simulink model "BLAC0_ControlloVelocitaNonCompensato"  (R2018b)
settings: Solver=ode1  StartTime=0.0  StopTime=0.1  FixedStep=1e-4  RelTol=1e-3
values from neighbouring files (symbols this model uses):
  B = 3.8e-005    (= 3.8e-05)    [BLAC0_v1.m]    (also in BLAC1_v1.m = 0; BLAC1_v2.m = 0; CAE_11_v_1.m = 0; CAE_14_v1.M = 0)
  J = 0.0000251    (= 2.51e-05)    [BLAC0_v1.m]    (also in BLAC1_v1.m = 0.001; BLAC1_v2.m = 0.001; CAE_11_v_1.m = 0.001; CAE_14_v1.M = 0.001)
  Kc = ms*np*lambdaf/2    (= 0.27)    [BLAC0_v1.m]    (also in BLAC1_v1.m = 0.6; BLAC1_v2.m = 0.6; CAE_11_v_1.m = 0.6; CAE_14_v1.M = 0.6)
  Lsd = 0.005/2    (= 0.0025)    [BLAC0_v1.m]    (also in BLAC1_v1.m = 0.005; BLAC1_v2.m = 0.005; CAE_11_v_1.m = 0.005; CAE_14_v1.M = 0.005)
  Lsq = Lsd    (= 0.0025)    [BLAC0_v1.m]    (also in BLAC1_v1.m = 0.005; BLAC1_v2.m = 0.005; CAE_11_v_1.m = 0.005; CAE_14_v1.M = 0.005)
  np = 2    [BLAC0_v1.m]    (also in BLAC1_v1.m = 4; BLAC1_v2.m = 4; CAE_11_v_1.m = 4; CAE_14_v1.M = 4)
  PSIPM = lambdaf    (= 0.09)    [BLAC0_v1.m]
  Rs = 3.1/2    (= 1.55)    [BLAC0_v1.m]    (also in BLAC1_v1.m = 1; BLAC1_v2.m = 1; CAE_11_v_1.m = 1; CAE_14_v1.M = 1)
  wrr = 1256.6    [BLAC0_v1.m]    (also in BLAC1_v1.m = 300; BLAC1_v2.m = 300)
settings Model: Creator=franc  LastModifiedBy=anton

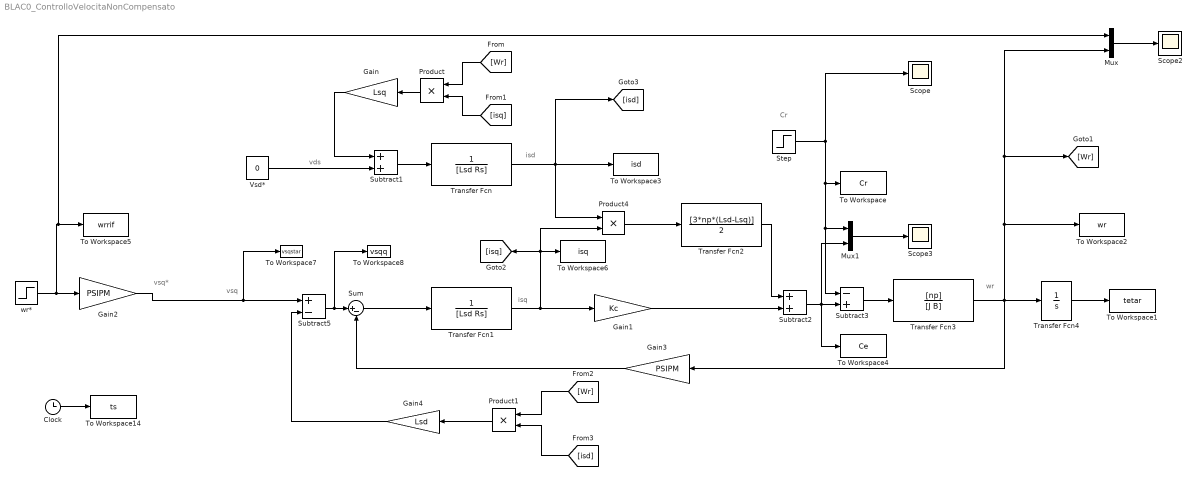
== system BLAC0_ControlloVelocitaNonCompensato ==
  note: isd
  note: isq
  note: wr
  note: vsq
  note: vsq*
  note: Cr
  note: vds
  Clock : Clock
  Gain : Gain  Gain=Lsq
  Gain1 : Gain  Gain=Kc
  Gain2 : Gain  Gain=PSIPM
  Gain3 : Gain  Gain=PSIPM
  Gain4 : Gain  Gain=Lsd
  Mux : Mux  Inputs=2
  Mux1 : Mux  Inputs=2
  Product : Product
  Product1 : Product
  Product4 : Product
  Scope : Scope
  Scope2 : Scope
  Scope3 : Scope
  Step : Step  Time=0.05  After=0.6  SampleTime=0
  Subtract1 : Sum
  Subtract2 : Sum
  Subtract3 : Sum  Inputs=-+
  Subtract5 : Sum  Inputs=+-
  Sum : Sum  Inputs=|+-
  To Workspace : ToWorkspace  VariableName=Cr  SampleTime=-1
  To Workspace1 : ToWorkspace  VariableName=tetar  SaveFormat=Timeseries  SampleTime=-1
  To Workspace14 : ToWorkspace  VariableName=ts  SampleTime=-1
  To Workspace2 : ToWorkspace  VariableName=wr  SampleTime=-1
  To Workspace3 : ToWorkspace  VariableName=isd  SaveFormat=Timeseries  SampleTime=-1
  To Workspace4 : ToWorkspace  VariableName=Ce  SampleTime=-1
  To Workspace5 : ToWorkspace  VariableName=wrrif  SampleTime=-1
  To Workspace6 : ToWorkspace  VariableName=isq  SaveFormat=Timeseries  SampleTime=-1
  To Workspace7 : ToWorkspace  VariableName=vsqstar  SampleTime=-1
  To Workspace8 : ToWorkspace  VariableName=vsqq  SampleTime=-1
  Transfer Fcn : TransferFcn  Denominator=[Lsd Rs]
  Transfer Fcn1 : TransferFcn  Denominator=[Lsd Rs]
  Transfer Fcn2 : TransferFcn  Numerator=[3*np*(Lsd-Lsq)]  Denominator=[2]
  Transfer Fcn3 : TransferFcn  Numerator=[np]  Denominator=[J B]
  Transfer Fcn4 : TransferFcn  Denominator=[1 0]
  Vsd* : Constant  Value=0
  wr* : Step  Time=0  After=wrr  SampleTime=0
  wires:
  Product/1 -> Gain/1
  Product4/1 -> Transfer Fcn2/1
  Subtract2/1 -> Mux1/2, Subtract3/2, To Workspace4/1
  Gain4/1 -> Subtract5/2
  Sum/1 -> Transfer Fcn1/1
  Transfer Fcn4/1 -> To Workspace1/1
  [isq] -> Product/2
  [Wr] -> Product/1
  Step/1 -> To Workspace/1, Mux1/1, Subtract3/1, Scope/1
  Transfer Fcn1/1 -> [isq], To Workspace6/1, Product4/2, Gain1/1
  Gain3/1 -> Sum/2
  Subtract5/1 -> To Workspace8/1, Sum/1
  Product1/1 -> Gain4/1
  Transfer Fcn/1 -> [isd], Product4/1, To Workspace3/1
  Transfer Fcn2/1 -> Subtract2/1
  Gain/1 -> Subtract1/1
  Subtract3/1 -> Transfer Fcn3/1
  Gain1/1 -> Subtract2/2
  [Wr] -> Product1/1
  Subtract1/1 -> Transfer Fcn/1
  Gain2/1 -> To Workspace7/1, Subtract5/1
  [isd] -> Product1/2
  Vsd*/1 -> Subtract1/2
  wr*/1 -> Mux/1, To Workspace5/1, Gain2/1
  Mux/1 -> Scope2/1
  Mux1/1 -> Scope3/1
  Transfer Fcn3/1 -> [Wr], Mux/2, To Workspace2/1, Transfer Fcn4/1, Gain3/1
  Clock/1 -> To Workspace14/1
